simulink model "tv_system_cordic"  (R2021b)
settings: Solver=VariableStepAuto  StartTime=0.0  StopTime=0  RelTol=1e-3
values from neighbouring files (symbols this model uses):
  gamma1 = 0.005    [main_pixloss.m]
  gamma2 = 1/(1.05*tau2)*(1/gamma1-beta/2)    [main_pixloss.m]
  lambda = 0.012    [main_pixloss.m]
  maxIter = 500    [main_pixloss.m]
undefined symbols (not defined in the file or in its folder): cols, rows
libraries: visionsources x3, visionstatistics x2
settings Model: Creator=abeshu  LastModifiedBy=shu_abe

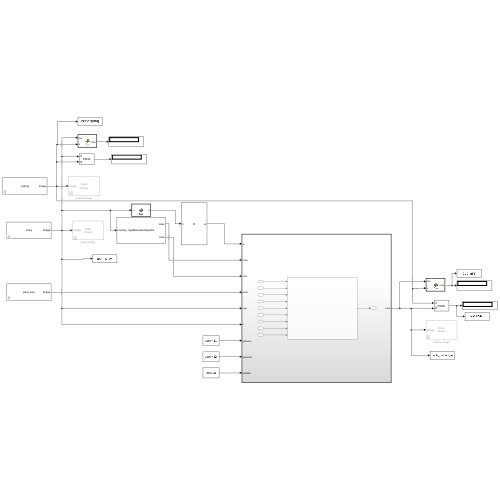
[thumbnail: Simulink's stored preview of the top-level diagram]
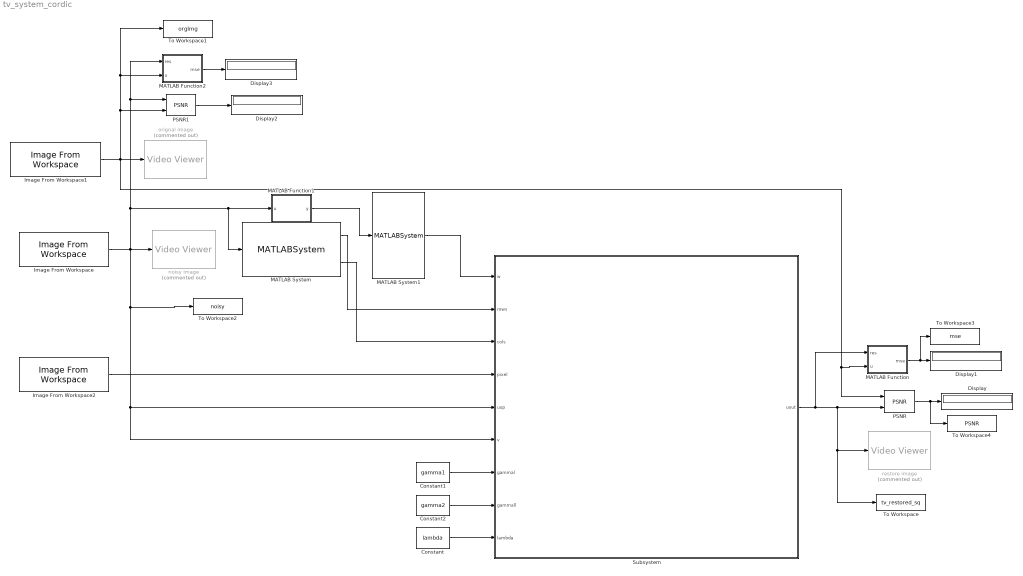
== system tv_system_cordic ==
  Constant : Constant  Value=lambda
  Constant1 : Constant  Value=gamma1
  Constant2 : Constant  Value=gamma2
  Display{,1..3} (4 alike) : Display
  Image From Workspace : visionsources/Image From Workspace  Tag=vipblks_nd  ImageValue=noisy  Ts=inf  imagePorts=One multidimensional signal  OutPortLabels=R|G|B  ImageDataType=Inherit from 'Value'  Signed=on  WordLength=16  sdImageDataType=sfix(16)  FractionLengthMode=User-defined  FractionLength=15
      settings: SourceProductBaseCode=VP
  Image From Workspace1 : visionsources/Image From Workspace  Tag=vipblks_nd  ImageValue=orgImg  Ts=inf  imagePorts=One multidimensional signal  OutPortLabels=R|G|B  ImageDataType=Inherit from 'Value'  Signed=on  WordLength=16  sdImageDataType=sfix(16)  FractionLengthMode=User-defined  FractionLength=15
      settings: SourceProductBaseCode=VP
  Image From Workspace2 : visionsources/Image From Workspace  Tag=vipblks_nd  ImageValue=pixel_loss  Ts=inf  imagePorts=One multidimensional signal  OutPortLabels=R|G|B  ImageDataType=Inherit from 'Value'  Signed=on  WordLength=16  sdImageDataType=sfix(16)  FractionLengthMode=User-defined  FractionLength=15
      settings: SourceProductBaseCode=VP
  MATLAB Function : MATLAB Function  TreatAsAtomicUnit=on
  MATLAB Function1 : MATLAB Function  TreatAsAtomicUnit=on
  MATLAB Function2 : MATLAB Function  TreatAsAtomicUnit=on
  MATLAB System : MATLABSystem  System=regObsevationSystem  SimulateUsing=Code generation
      mask Type: regObsevationSystem
      mask Display:
      | disp('regObsevationSystem');
      | port_label('input',1,'imnoisy');
      | port_label('output',1,'rows');
      | port_label('output',2,'colw');
  MATLAB System1 : MATLABSystem  System=dBlockSystem  SimulateUsing=Code generation
      mask Type: dBlockSystem
      mask Display:
      | disp('D');
      | port_label('input',1,'z');
      | port_label('output',1,'w');
  PSNR : visionstatistics/PSNR
      settings: SourceProductBaseCode=VP
  PSNR1 : visionstatistics/PSNR
      settings: SourceProductBaseCode=VP
  Subsystem : Subsystem  TreatAsAtomicUnit=on
  To Workspace : ToWorkspace  VariableName=tv_restored_sq  SaveFormat=Structure  SampleTime=-1
      settings: Save2DSignal=2-D array (concatenate along first dimension)
  To Workspace1 : ToWorkspace  VariableName=orgImg  SaveFormat=Structure  SampleTime=-1
      settings: Save2DSignal=2-D array (concatenate along first dimension)
  To Workspace2 : ToWorkspace  VariableName=noisy  SaveFormat=Structure  SampleTime=-1
      settings: Save2DSignal=2-D array (concatenate along first dimension)
  To Workspace3 : ToWorkspace  VariableName=mse  SaveFormat=Structure  SampleTime=-1
      settings: Save2DSignal=2-D array (concatenate along first dimension)
  To Workspace4 : ToWorkspace  VariableName=PSNR  SaveFormat=Structure  SampleTime=-1
      settings: Save2DSignal=2-D array (concatenate along first dimension)
  noisy image : VideoViewer  Commented=on  FigPos=[349 887 308 381]
  orignal image : VideoViewer  Commented=on  FigPos=[248 697 520 310]
  restore image : VideoViewer  Commented=on  FigPos=[19 892 539 328]
  wires:
  Image From Workspace/1 -> To Workspace2/1, Subsystem/6(v), Subsystem/5(uup), MATLAB Function2/1(res), PSNR1/1, MATLAB System/1, MATLAB Function1/1(u), noisy image/1
  Image From Workspace1/1 -> To Workspace1/1, MATLAB Function2/2(u), PSNR1/2, MATLAB Function/2(u), PSNR/1, orignal image/1
  Image From Workspace2/1 -> Subsystem/4(pixel)
  MATLAB System/1 -> Subsystem/2(rows)
  MATLAB System/2 -> Subsystem/3(cols)
  MATLAB Function1/1(y) -> MATLAB System1/1
  Constant1/1 -> Subsystem/7(gammal)
  Constant2/1 -> Subsystem/8(gammall)
  Constant/1 -> Subsystem/9(lambda)
  MATLAB System1/1 -> Subsystem/1(w)
  Subsystem/1(uout) -> To Workspace/1, restore image/1, PSNR/2, MATLAB Function/1(res)
  PSNR/1 -> To Workspace4/1, Display/1
  MATLAB Function/1(mse) -> To Workspace3/1, Display1/1
  PSNR1/1 -> Display2/1
  MATLAB Function2/1(mse) -> Display3/1

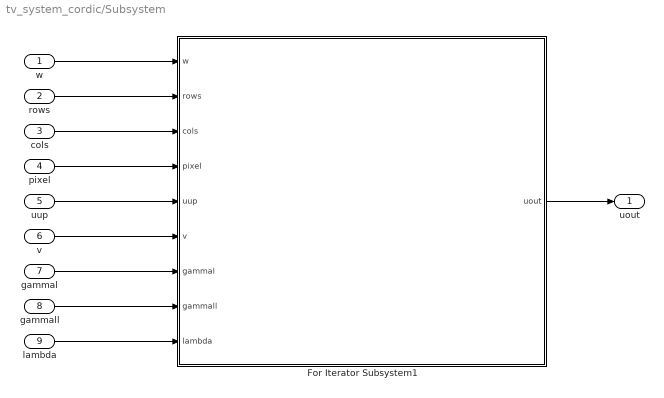
== system tv_system_cordic/Subsystem ==
  w : Inport
  rows : Inport  Port=2
  cols : Inport  Port=3
  pixel : Inport  Port=4
  uup : Inport  Port=5
  v : Inport  Port=6
  gammal : Inport  Port=7
  gammall : Inport  Port=8
  lambda : Inport  Port=9
  For Iterator Subsystem1 : Subsystem  TreatAsAtomicUnit=on
  uout : Outport
  wires:
  For Iterator Subsystem1/1(uout) -> uout/1
  w/1 -> For Iterator Subsystem1/1(w)
  rows/1 -> For Iterator Subsystem1/2(rows)
  cols/1 -> For Iterator Subsystem1/3(cols)
  pixel/1 -> For Iterator Subsystem1/4(pixel)
  uup/1 -> For Iterator Subsystem1/5(uup)
  v/1 -> For Iterator Subsystem1/6(v)
  gammal/1 -> For Iterator Subsystem1/7(gammal)
  gammall/1 -> For Iterator Subsystem1/8(gammall)
  lambda/1 -> For Iterator Subsystem1/9(lambda)

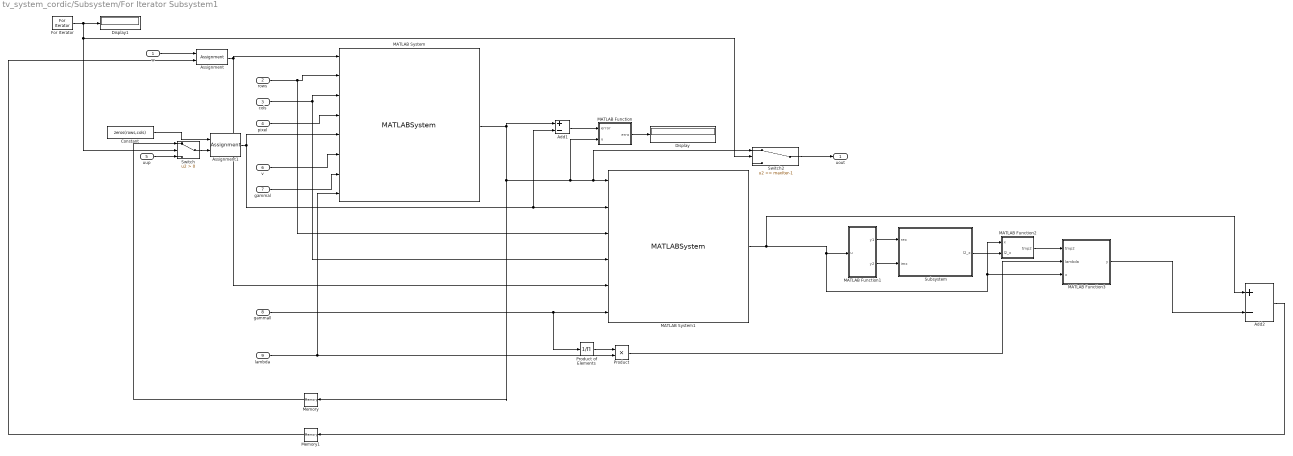
== system tv_system_cordic/Subsystem/For Iterator Subsystem1 ==
  w : Inport
  rows : Inport  Port=2
  cols : Inport  Port=3
  pixel : Inport  Port=4
  uup : Inport  Port=5
  v : Inport  Port=6
  gammal : Inport  Port=7
  gammall : Inport  Port=8
  lambda : Inport  Port=9
  Add1 : Sum  Inputs=+-
  Add2 : Sum  Inputs=+-
  Assignment : Assignment  NumberOfDimensions=3  DiagnosticForDimensions=Warning  IndexOptions=Assign all,Assign all,Assign all  Indices=1,1,1  OutputSizes=1,1,1
  Assignment1 : Assignment  NumberOfDimensions=2  DiagnosticForDimensions=Warning  IndexOptions=Assign all,Assign all  Indices=1,1  OutputSizes=1,1
  Constant : Constant  Value=zeros(rows,cols)
  Display : Display
  Display1 : Display
  For Iterator : ForIterator  IterationLimit=maxIter  IndexMode=Zero-based  IterationVariableDataType=double
  MATLAB Function : MATLAB Function  TreatAsAtomicUnit=on
  MATLAB Function1 : MATLAB Function  TreatAsAtomicUnit=on
  MATLAB Function2 : MATLAB Function  TreatAsAtomicUnit=on
  MATLAB Function3 : MATLAB Function  TreatAsAtomicUnit=on
  MATLAB System : MATLABSystem  System=updateuSystem  SimulateUsing=Code generation
      mask Type: updateuSystem
      mask Display:
      | disp('updateuSystem');
      | port_label('input',1,'w');
      | port_label('input',2,'rows');
      | port_label('input',3,'cols');
      | port_label('input',4,'pixel');
      | port_label('input',5,'uup');
      | port_label('input',6,'v');
      | port_label('input',7,'gamma1');
      | port_label('input',8,'lambda');
      | port_label('output',1,'u');
  MATLAB System1 : MATLABSystem  System=updatewSystem  SimulateUsing=Code generation
      mask Type: updatewSystem
      mask Display:
      | disp('updatewSystem');
      | port_label('input',1,'u');
      | port_label('input',2,'upre');
      | port_label('input',3,'rows');
      | port_label('input',4,'cols');
      | port_label('input',5,'w');
      | port_label('input',6,'gamma2');
      | port_label('output',1,'w_tilde');
  Memory : Memory  InheritSampleTime=on
  Memory1 : Memory  InheritSampleTime=on
  Product : Product
  Product of Elements : Product  Inputs=/
  Subsystem : Subsystem
  Switch : Switch  Criteria=u2 > Threshold
  Switch2 : Switch  Threshold=maxIter-1
  uout : Outport
  wires:
  w/1 -> Assignment/1
  Assignment/1 -> MATLAB System/1, MATLAB System1/5
  rows/1 -> MATLAB System/2, MATLAB System1/3
  cols/1 -> MATLAB System1/4, MATLAB System/3
  pixel/1 -> MATLAB System/4
  Constant/1 -> Assignment1/1
  Switch/1 -> Assignment1/2
  uup/1 -> Switch/3
  Assignment1/1 -> Add1/2, MATLAB System1/2, MATLAB System/5
  v/1 -> MATLAB System/6
  gammal/1 -> MATLAB System/7
  For Iterator/1 -> Switch/2, Switch2/2, Display1/1
  MATLAB System/1 -> Add1/1, Switch2/1, MATLAB System1/1, MATLAB Function/2(u), Memory/1
  Add1/1 -> MATLAB Function/1(error)
  MATLAB Function/1(erro) -> Display/1
  gammall/1 -> Product of Elements/1, MATLAB System1/6
  MATLAB Function1/1(y1) -> Subsystem/1(rex)
  MATLAB System1/1 -> MATLAB Function3/3(x), MATLAB Function2/1(x), MATLAB Function1/1(u), Add2/1
  Subsystem/1(l2_x) -> MATLAB Function2/2(l2_x)
  MATLAB Function2/1(tmp2) -> MATLAB Function3/1(tmp2)
  Product of Elements/1 -> Product/1
  lambda/1 -> MATLAB System/8, Product/2
  Product/1 -> MATLAB Function3/2(lambda)
  Memory/1 -> Switch/1
  Add2/1 -> Memory1/1
  MATLAB Function3/1(y) -> Add2/2
  Memory1/1 -> Assignment/2
  Switch2/1 -> uout/1
  MATLAB Function1/2(y2) -> Subsystem/2(imx)

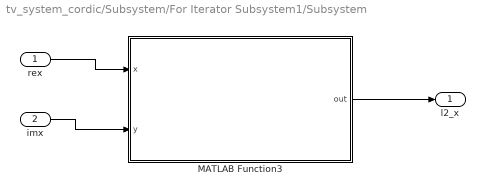
== system tv_system_cordic/Subsystem/For Iterator Subsystem1/Subsystem ==
  rex : Inport
  imx : Inport  Port=2
  MATLAB Function3 : MATLAB Function  TreatAsAtomicUnit=on
  l2_x : Outport
  wires:
  rex/1 -> MATLAB Function3/1(x)
  imx/1 -> MATLAB Function3/2(y)
  MATLAB Function3/1(out) -> l2_x/1

== matlab function tv_system_cordic/MATLAB Function ==
  data: res input; u input; mse output
function mse = fcn(res,u)

mse = immse(u,res);

== matlab function tv_system_cordic/Subsystem/For Iterator Subsystem1/MATLAB Function ==
  data: error input; u input; erro output
function erro = fcn(error,u)

erro = norm(error(:),2) / norm(u(:),2);

== matlab function tv_system_cordic/MATLAB Function2 ==
  data: res input; u input; mse output
function mse = fcn(res,u)

mse = immse(u,res);

== matlab function tv_system_cordic/Subsystem/For Iterator Subsystem1/MATLAB Function1 ==
  data: u input; y1 output; y2 output
function [y1,y2] = fcn(u)
    y1 = u(:,:,1);
    y2 = u(:,:,2);
end

== matlab function tv_system_cordic/Subsystem/For Iterator Subsystem1/MATLAB Function2 ==
  data: x input; tmp2 output; l2_x input
function tmp2 = fcn(x,l2_x)

if isfi(x) == true
    tmp2 = divide(x.numerictype,1,l2_x);
else
    tmp2 = 1./l2_x;
end

== matlab function tv_system_cordic/Subsystem/For Iterator Subsystem1/MATLAB Function3 ==
  data: tmp2 input; y output; lambda input; x input
function y = fcn(tmp2,lambda,x)

% tmp3 = lambda*tmp2;
y = repmat(max(1 - tmp2,0),1,1,2) .* x;

== matlab function tv_system_cordic/Subsystem/For Iterator Subsystem1/Subsystem/MATLAB Function3 ==
  data: x input; out output; y input
function out = l2_cordic(x,y)

tmp1 = x.^2 + y.^2;
tmp1 = cast(tmp1,'like',x);
out = cordicsqrt(tmp1);

end

== matlab function tv_system_cordic/MATLAB Function1 ==
  data: u input; y output
function y = fcn(u)

y = zeros(size(u));
